simulink model "BO_diag"  (R2024b)
settings: Solver=VariableStepAuto  StartTime=0.0  StopTime=10.0  RelTol=1e-3
values from neighbouring files (symbols this model uses):
  plant_ss_diag = diagonalize(plant_ss)    [Copy_of_main_final.m]    (also in diagonalize.m = ss(A_d, B_d, C_d, 0))
settings Model: Creator=dsagn  LastModifiedBy=dsagn

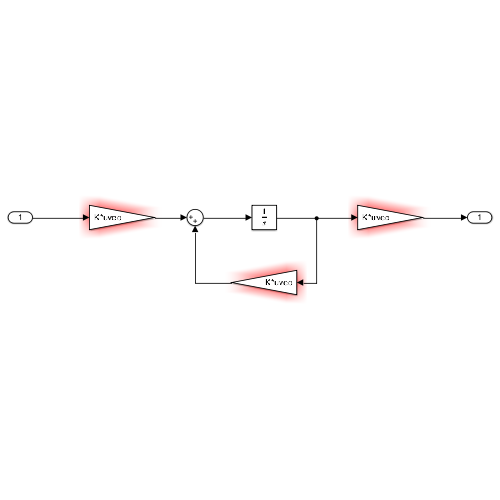
[thumbnail: Simulink's stored preview of the top-level diagram]
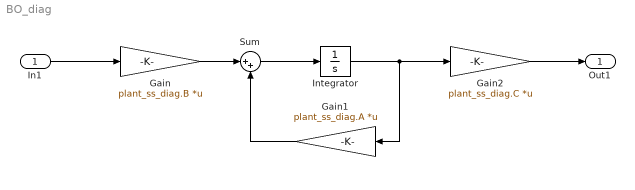
== system BO_diag ==
  In1 : Inport
  Gain : Gain  Gain=plant_ss_diag.B  Multiplication=Matrix(K*u) (u vector)
  Gain1 : Gain  Gain=plant_ss_diag.A  Multiplication=Matrix(K*u) (u vector)
  Gain2 : Gain  Gain=plant_ss_diag.C  Multiplication=Matrix(K*u) (u vector)
  Integrator : Integrator
  Sum : Sum  Inputs=|++
  Out1 : Outport
  wires:
  Sum/1 -> Integrator/1
  Integrator/1 -> Gain1/1, Gain2/1
  Gain1/1 -> Sum/2
  Gain/1 -> Sum/1
  In1/1 -> Gain/1
  Gain2/1 -> Out1/1
